simulink model "ThreeToEightDecoder"  (R2017b)
settings: Solver=VariableStepAuto  StartTime=0.0  StopTime=10.0  RelTol=1e-3
settings Model: Creator=Ray  LastModifiedBy=Ray

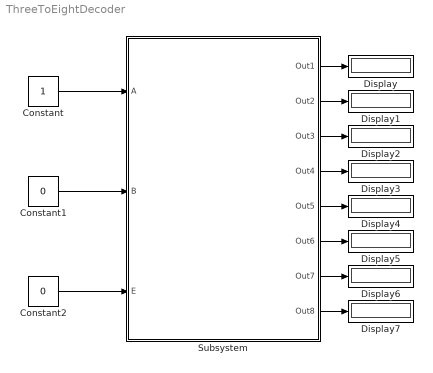
== system ThreeToEightDecoder ==
  Constant : Constant  OutDataTypeStr=boolean  SampleTime=1
  Constant1 : Constant  Value=0  OutDataTypeStr=boolean  SampleTime=1
  Constant2 : Constant  Value=0  OutDataTypeStr=boolean  SampleTime=1
  Display{,1..7} (8 alike) : Display
  Subsystem : Subsystem
  wires:
  Subsystem/1(Out1) -> Display/1
  Subsystem/2(Out2) -> Display1/1
  Subsystem/3(Out3) -> Display2/1
  Subsystem/4(Out4) -> Display3/1
  Subsystem/5(Out5) -> Display4/1
  Subsystem/6(Out6) -> Display5/1
  Subsystem/7(Out7) -> Display6/1
  Subsystem/8(Out8) -> Display7/1
  Constant/1 -> Subsystem/1(A)
  Constant1/1 -> Subsystem/2(B)
  Constant2/1 -> Subsystem/3(E)

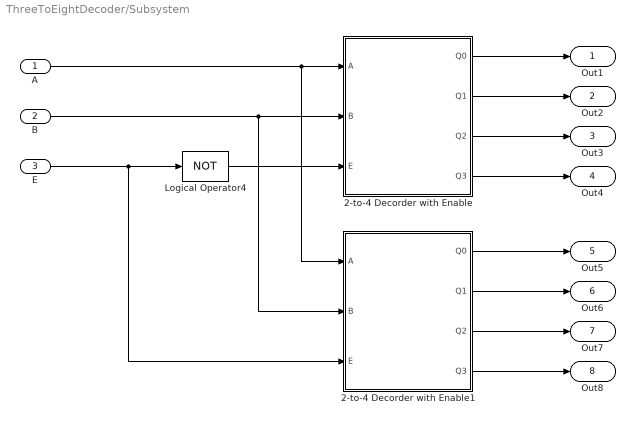
== system ThreeToEightDecoder/Subsystem ==
  A : Inport  OutDataTypeStr=boolean  SampleTime=1
  B : Inport  Port=2  OutDataTypeStr=boolean  SampleTime=1
  E : Inport  Port=3  OutDataTypeStr=boolean  SampleTime=1
  2-to-4 Decorder with Enable : Subsystem
  2-to-4 Decorder with Enable1 : Subsystem
  Logical Operator4 : Logic  Operator=NOT  Inputs=3  IconShape=distinctive  AllPortsSameDT=off  OutDataTypeStr=boolean
  Out1 : Outport  OutDataTypeStr=boolean  SampleTime=1
  Out2 : Outport  Port=2  OutDataTypeStr=boolean  SampleTime=1
  Out3 : Outport  Port=3  OutDataTypeStr=boolean  SampleTime=1
  Out4 : Outport  Port=4  OutDataTypeStr=boolean  SampleTime=1
  Out5 : Outport  Port=5  OutDataTypeStr=boolean  SampleTime=1
  Out6 : Outport  Port=6  OutDataTypeStr=boolean  SampleTime=1
  Out7 : Outport  Port=7  OutDataTypeStr=boolean  SampleTime=1
  Out8 : Outport  Port=8  OutDataTypeStr=boolean  SampleTime=1
  wires:
  2-to-4 Decorder with Enable/3(Q2) -> Out3/1
  2-to-4 Decorder with Enable1/2(Q1) -> Out6/1
  2-to-4 Decorder with Enable/2(Q1) -> Out2/1
  2-to-4 Decorder with Enable1/3(Q2) -> Out7/1
  2-to-4 Decorder with Enable1/1(Q0) -> Out5/1
  2-to-4 Decorder with Enable/1(Q0) -> Out1/1
  2-to-4 Decorder with Enable1/4(Q3) -> Out8/1
  2-to-4 Decorder with Enable/4(Q3) -> Out4/1
  Logical Operator4/1 -> 2-to-4 Decorder with Enable/3(E)
  E/1 -> Logical Operator4/1, 2-to-4 Decorder with Enable1/3(E)
  B/1 -> 2-to-4 Decorder with Enable1/2(B), 2-to-4 Decorder with Enable/2(B)
  A/1 -> 2-to-4 Decorder with Enable1/1(A), 2-to-4 Decorder with Enable/1(A)

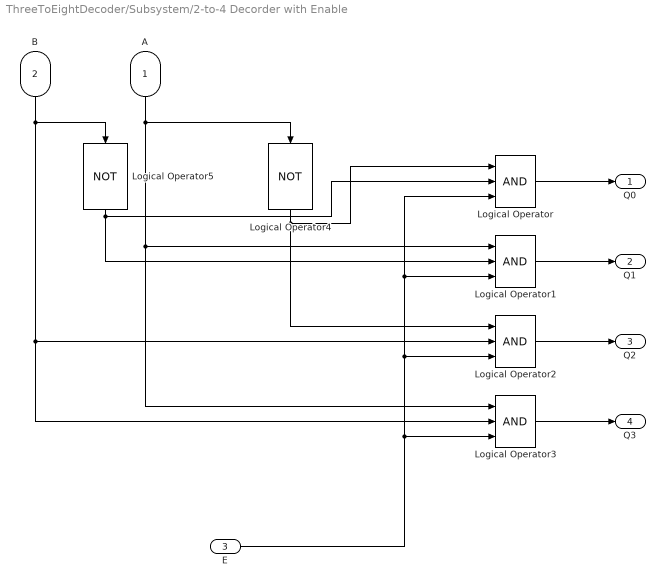
== system ThreeToEightDecoder/Subsystem/2-to-4 Decorder with Enable ==
  A : Inport  OutDataTypeStr=boolean  SampleTime=1
  B : Inport  Port=2  OutDataTypeStr=boolean  SampleTime=1
  E : Inport  Port=3  OutDataTypeStr=boolean  SampleTime=1
  Logical Operator{,1..3} (4 alike) : Logic  Inputs=3  IconShape=distinctive  AllPortsSameDT=off  OutDataTypeStr=boolean
  Logical Operator4 : Logic  Operator=NOT  Inputs=3  IconShape=distinctive  AllPortsSameDT=off  OutDataTypeStr=boolean
  Logical Operator5 : Logic  Operator=NOT  Inputs=3  IconShape=distinctive  AllPortsSameDT=off  OutDataTypeStr=boolean
  Q0 : Outport  SampleTime=1
  Q1 : Outport  Port=2  SampleTime=1
  Q2 : Outport  Port=3  SampleTime=1
  Q3 : Outport  Port=4  SampleTime=1
  wires:
  Logical Operator5/1 -> Logical Operator1/2, Logical Operator/2
  Logical Operator2/1 -> Q2/1
  Logical Operator4/1 -> Logical Operator2/1, Logical Operator/1
  Logical Operator3/1 -> Q3/1
  Logical Operator1/1 -> Q1/1
  Logical Operator/1 -> Q0/1
  A/1 -> Logical Operator1/1, Logical Operator3/1, Logical Operator4/1
  B/1 -> Logical Operator2/2, Logical Operator3/2, Logical Operator5/1
  E/1 -> Logical Operator3/3, Logical Operator2/3, Logical Operator1/3, Logical Operator/3

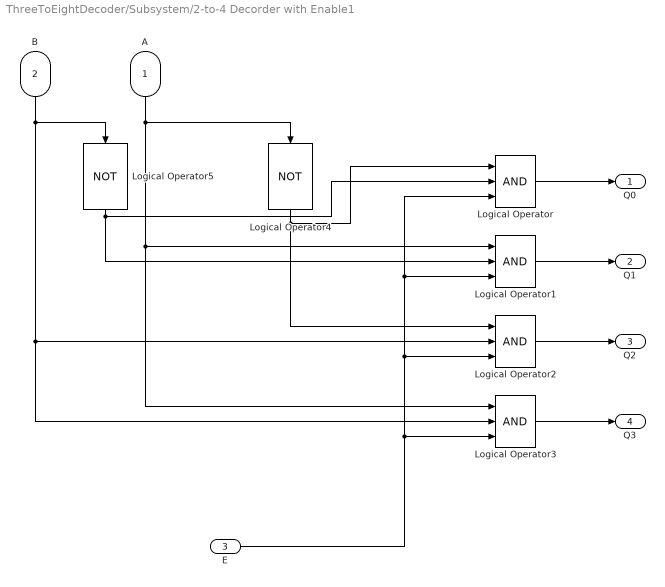
== system ThreeToEightDecoder/Subsystem/2-to-4 Decorder with Enable1 ==
  A : Inport  OutDataTypeStr=boolean  SampleTime=1
  B : Inport  Port=2  OutDataTypeStr=boolean  SampleTime=1
  E : Inport  Port=3  OutDataTypeStr=boolean  SampleTime=1
  Logical Operator{,1..3} (4 alike) : Logic  Inputs=3  IconShape=distinctive  AllPortsSameDT=off  OutDataTypeStr=boolean
  Logical Operator4 : Logic  Operator=NOT  Inputs=3  IconShape=distinctive  AllPortsSameDT=off  OutDataTypeStr=boolean
  Logical Operator5 : Logic  Operator=NOT  Inputs=3  IconShape=distinctive  AllPortsSameDT=off  OutDataTypeStr=boolean
  Q0 : Outport  SampleTime=1
  Q1 : Outport  Port=2  SampleTime=1
  Q2 : Outport  Port=3  SampleTime=1
  Q3 : Outport  Port=4  SampleTime=1
  wires:
  Logical Operator5/1 -> Logical Operator1/2, Logical Operator/2
  Logical Operator2/1 -> Q2/1
  Logical Operator4/1 -> Logical Operator2/1, Logical Operator/1
  Logical Operator3/1 -> Q3/1
  Logical Operator1/1 -> Q1/1
  Logical Operator/1 -> Q0/1
  A/1 -> Logical Operator1/1, Logical Operator3/1, Logical Operator4/1
  B/1 -> Logical Operator2/2, Logical Operator3/2, Logical Operator5/1
  E/1 -> Logical Operator3/3, Logical Operator2/3, Logical Operator1/3, Logical Operator/3
